simulink model "Model_plane2_Oldvers"  (R2023b)
settings: Solver=VariableStepAuto  StartTime=0.0  StopTime=5.0  RelTol=1e-3
values from neighbouring files (symbols this model uses):
  a_table = [340.3 339.5 338.8 338.0 337.2 336.4]    [Table1.m]
  Alfa = [-2 4 10 16]    [Table1.m]
  Alfa_table = [-4 0 5 10 20]    [Table1.m]
  Alfa_y = [-4 6 8 9 10 12 14]    [Table1.m]
  Cxa_table = [0.03434 0.0358 0.04274 ... (first row only)    [Table1.m]
  Cy_DB = [0.01242 0.01286 0.01457]    [Table1.m]
  Cy_fi = [0.00623 0.00643 0.00626]    [Table1.m]
  Cya = [-0.276 -0.330 -0.390 ... (first row only)    [Table1.m]
  H = [339 3256 4060 8000 12000]    [Table1.m]
  H_table = 0:2000:10000    [Table1.m]
  M_C = [0.4 0.6 0.82]    [Table1.m]
  M_mz = [0.2 0.4 0.6 0.8]    [Table1.m]
  M_mz2 = [0.4 0.7 0.85]    [Table1.m]
  M_table = [0.4 0.7 0.82]    [Table1.m]
  M_y = [0.4 0.7 0.82]    [Table1.m]
  mz_alfa = [-0.0282 -0.0282 -0.0289 -0.0404]    [Table1.m]
  mz_alfa2 = [-8.163 -8.762 -9.714 ... (first row only)    [Table1.m]
  mz_DB = [-0.0350 -0.0358 -0.0370 -0.0377]    [Table1.m]
  mz_fi = [-0.0695 -0.0714 -0.0739 -0.0832]    [Table1.m]
  mz_omz = [-23.768 -25.300 -28.284 ... (first row only)    [Table1.m]
  P = [9088 7396 6783 5000 4000]    [Table1.m]
  q_table = [1.225 1.2017 1.1786 1.1560 1.1337 1.1117]    [Table1.m]
libraries: simulink x2
settings Model: Creator=Анастасия  LastModifiedBy=Анастасия
settings RTWCC: GPUComputeCapability=5.0

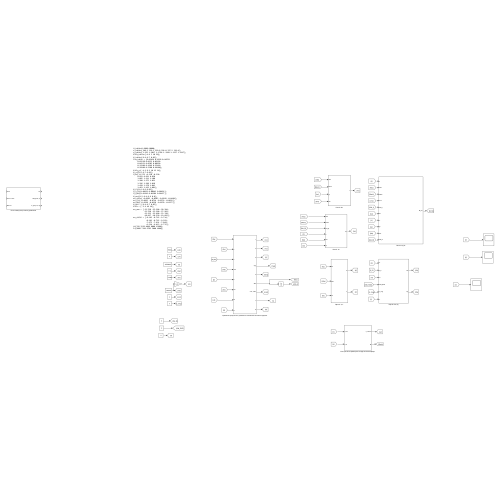
[thumbnail: Simulink's stored preview of the top-level diagram]
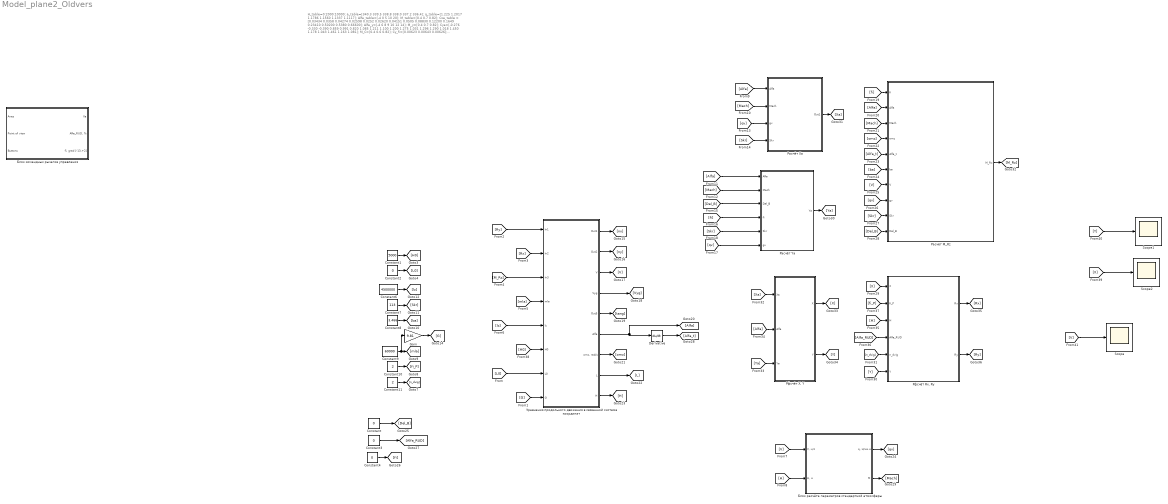
== system Model_plane2_Oldvers ==
  note: H_table=0:2000:10000;
      | a_table=[340.3 339.5 338.8 338.0 337.2 336.4];
      | q_table=[1.225 1.2017 1.1786 1.1560 1.1337 1.1117];
      | Alfa_table=[-4 0 5 10 20];
      | M_table=[0.4 0.7 0.82];
      | Cxa_table = [0.03434 0.0358 0.04274
      | 0.02598 0.0252 0.02620
      | 0.04151 0.0505 0.08830
      | 0.12200 0.1649 0.23410
      | 0.50200 0.5380 0.66600];
      | Alfa_y=[-4 6 8 9 10 12 14];
      | M_y=[0.4 0.7 0.82];
      | Cya=[-0.276 -0.330 -0.390
      | 0.859 0.991 0.820
      | 1.085 1.211 1.100
      | 1.200 1.275 1.031
      | 1.296 1.290 1.018
      | 1.450 1.178 1.043
      | 1.461 1.163 1.081];
      | M_C=[0.4 0.6 0.82];
      | Cy_fi=[0.00623 0.00643 0.00626];
      | Cy_DB=[0.01242 0.01286 0.01457];
      | M_mz=[0.2 0.4 0.6 0.8];
      | mz_alfa=[-0.0282 -0.0282 -0.0289 -0.0404];
      | mz_fi=[-0.0695 -0.0714 -0.0739 -0.0832];
      | mz_DB=[-0.0350 -0.0358 -0.0370 -0.0377];
      | M_mz2 = [0.4 0.7 0.85];
      | Alfa = [-2 4 10 16];
      | mz_omz = [-23.768 -25.300 -28.284;
      | -23.768 -25.300 -27.903;
      | -23.222 -22.600 -23.320;
      | -18.967 -18.520 -19.601];
      | mz_alfa2 = [-8.163 -8.762 -9.714;
      | -8.163 -8.762 -9.583;
      | -7.975 -7.991 -7.868;
      | -6.514 -6.413 -6.732];
      | H=[339 3256 4060 8000 12000];
      | P=[9088 7396 6783 5000 4000];
  Constant{,2..4} (4 alike) : Constant  Value=0
  Constant1 : Constant  Value=5000
  Constant10 : Constant  Value=2
  Constant11 : Constant  Value=2
  Constant6 : Constant  Value=4500000
  Constant7 : Constant  Value=113
  Constant8 : Constant  Value=3.466
  Constant9 : Constant  Value=60000
  Derivative : Derivative
  Gain : Gain  Gain=9.81
  Scope : Scope
  Scope1 : Scope
  Scope2 : Scope
  Блок командных рычагов управления : Subsystem
  Блок расчёта параметров стандартной атмосферы : Subsystem
  Расчёт M_Rz : Subsystem
  Расчёт Xa : Subsystem
  Расчёт Ya : Subsystem
  "Рфсчёт Rx, Ry" : Subsystem
  "Рфсчёт X, Y" : Subsystem
  Уравнения продольного движения в связанной системе координат : Subsystem
  wires:
  Constant1/1 -> [H0]
  Constant2/1 -> [L0]
  Constant6/1 -> [lz]
  Constant7/1 -> [Skr]
  Constant8/1 -> [ba]
  Constant9/1 -> Gain/1, [mla]
  Constant10/1 -> [fi_P]
  Constant11/1 -> [n_dvig]
  Gain/1 -> [G]
  [Ry] -> Уравнения продольного движения в связанной системе координат/1(In1)
  [Rx] -> Уравнения продольного движения в связанной системе координат/2(In2)
  [M_Rz] -> Уравнения продольного движения в связанной системе координат/3(In3)
  [mla] -> Уравнения продольного движения в связанной системе координат/4(mla)
  [lz] -> Уравнения продольного движения в связанной системе координат/5(lz)
  Уравнения продольного движения в связанной системе координат/1(Out1) -> [nx]
  Уравнения продольного движения в связанной системе координат/2(Out2) -> [ny]
  Уравнения продольного движения в связанной системе координат/3(V) -> [V]
  Уравнения продольного движения в связанной системе координат/4(Vyg) -> [Vyg]
  Уравнения продольного движения в связанной системе координат/5(Out5) -> [tang]
  Уравнения продольного движения в связанной системе координат/6(Alfa) -> Derivative/1, [Alfa]
  Уравнения продольного движения в связанной системе координат/7("omz, rad/s") -> [omz]
  Уравнения продольного движения в связанной системе координат/8(L) -> [L]
  Уравнения продольного движения в связанной системе координат/9(H) -> [H]
  Derivative/1 -> [Alfa_t]
  [V] -> Блок расчёта параметров стандартной атмосферы/1("V, м/с")
  [H] -> Блок расчёта параметров стандартной атмосферы/2("H, м")
  Блок расчёта параметров стандартной атмосферы/1("q, Н/кв.м") -> [qv]
  Блок расчёта параметров стандартной атмосферы/2(М) -> [Mach]
  [Alfa] -> Расчёт Xa/1(Alfa)
  [Mach] -> Расчёт Xa/2(Mach)
  [Mach] -> Расчёт Ya/2(Mach)
  [Alfa] -> Расчёт Ya/1(Alfa)
  Расчёт Xa/1(Out1) -> [Xa]
  Расчёт Ya/1(Ya) -> [Ya]
  [Skr] -> Расчёт Xa/4(Skr)
  [qv] -> Расчёт Xa/3(gv)
  [Del_B] -> Расчёт Ya/3(Del_B)
  [fi] -> Расчёт Ya/4(fi)
  [qv] -> Расчёт Ya/6(gv)
  [Skr] -> Расчёт Ya/5(Skr)
  Расчёт M_Rz/1(M_Rz) -> [M_Rz]
  [fi] -> Расчёт M_Rz/1(fi)
  [Alfa] -> Расчёт M_Rz/2(Alfa)
  [omz] -> Расчёт M_Rz/4(omz)
  [Mach] -> Расчёт M_Rz/3(Mach)
  [Alfa_t] -> Расчёт M_Rz/5(Alfa_t)
  [ba] -> Расчёт M_Rz/6(ba)
  [qv] -> Расчёт M_Rz/8(gv)
  [Del_B] -> Расчёт M_Rz/10(Del_B)
  [Skr] -> Расчёт M_Rz/9(Skr)
  [V] -> Расчёт M_Rz/7(V)
  "Рфсчёт X, Y"/1(X) -> [X]
  "Рфсчёт X, Y"/2(Y) -> [Y]
  [X] -> "Рфсчёт Rx, Ry"/1(X)
  [Y] -> "Рфсчёт Rx, Ry"/6(Y)
  "Рфсчёт Rx, Ry"/1(Rx) -> [Rx]
  "Рфсчёт Rx, Ry"/2(Ry) -> [Ry]
  [Xa] -> "Рфсчёт X, Y"/1(Xa)
  [Ya] -> "Рфсчёт X, Y"/3(Ya)
  [Alfa] -> "Рфсчёт X, Y"/2(Alfa)
  [Alfa_RUD] -> "Рфсчёт Rx, Ry"/4(Alfa_RUD)
  [n_dvig] -> "Рфсчёт Rx, Ry"/5(n_dvig)
  [H] -> "Рфсчёт Rx, Ry"/3(H)
  [fi_P] -> "Рфсчёт Rx, Ry"/2(fi_P)
  [H0] -> Уравнения продольного движения в связанной системе координат/6(H0)
  [L0] -> Уравнения продольного движения в связанной системе координат/7(L0)
  [G] -> Уравнения продольного движения в связанной системе координат/8(G)
  [V] -> Scope/1
  Constant4/1 -> [fi]
  Constant3/1 -> [Alfa_RUD]
  Constant/1 -> [Del_B]
  [Y] -> Scope1/1
  [X] -> Scope2/1

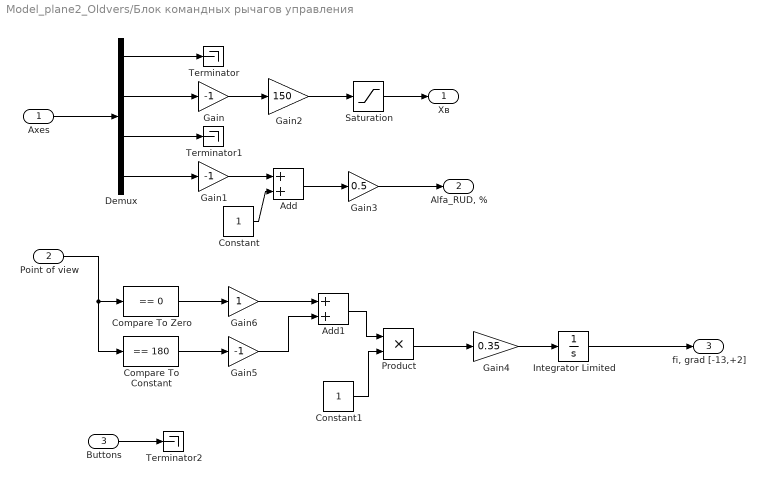
== system Model_plane2_Oldvers/Блок командных рычагов управления ==
  Axes : Inport
  Point of view : Inport  Port=2
  Buttons : Inport  Port=3
  Add : Sum
  Add1 : Sum
  Compare To Constant : simulink/Logic and Bit Operations/Compare To Constant  relop===  const=180  OutDataTypeStr=boolean
  Compare To Zero : simulink/Logic and Bit Operations/Compare To Zero  relop===  OutDataTypeStr=boolean
  Constant : Constant
  Constant1 : Constant
  Demux : Demux
  Gain : Gain  Gain=-1
  Gain1 : Gain  Gain=-1
  Gain2 : Gain  Gain=150
  Gain3 : Gain  Gain=0.5
  Gain4 : Gain  Gain=0.35
  Gain5 : Gain  Gain=-1
  Gain6 : Gain
  Integrator Limited : Integrator  LimitOutput=on  UpperSaturationLimit=1  LowerSaturationLimit=0
  Product : Product
  Saturation : Saturate
  Terminator : Terminator
  Terminator1 : Terminator
  Terminator2 : Terminator
  Xв : Outport
  "Alfa_RUD, %" : Outport  Port=2
  "fi, grad [-13,+2]" : Outport  Port=3
  wires:
  Axes/1 -> Demux/1
  Demux/1 -> Terminator/1
  Demux/3 -> Terminator1/1
  Demux/2 -> Gain/1
  Gain/1 -> Gain2/1
  Gain2/1 -> Saturation/1
  Saturation/1 -> Xв/1
  Demux/4 -> Gain1/1
  Gain1/1 -> Add/1
  Constant/1 -> Add/2
  Add/1 -> Gain3/1
  Gain3/1 -> "Alfa_RUD, %"/1
  Integrator Limited/1 -> "fi, grad [-13,+2]"/1
  Gain4/1 -> Integrator Limited/1
  Product/1 -> Gain4/1
  Constant1/1 -> Product/2
  Add1/1 -> Product/1
  Gain5/1 -> Add1/2
  Gain6/1 -> Add1/1
  Compare To Zero/1 -> Gain6/1
  Compare To Constant/1 -> Gain5/1
  Point of view/1 -> Compare To Constant/1, Compare To Zero/1
  Buttons/1 -> Terminator2/1

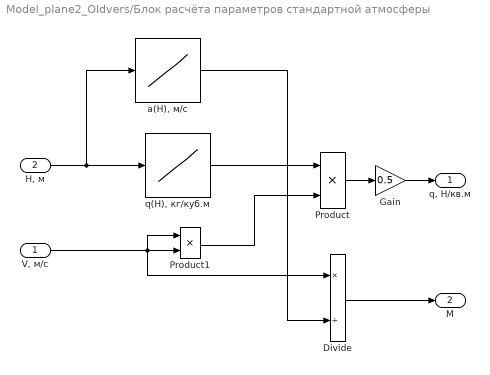
== system Model_plane2_Oldvers/Блок расчёта параметров стандартной атмосферы ==
  "V, м/с" : Inport
  "H, м" : Inport  Port=2
  Divide : Product  Inputs=*/
  Gain : Gain  Gain=0.5
  Product : Product
  Product1 : Product
  "a(H), м/с" : Lookup_n-D  NumberOfTableDimensions=1  BreakpointsForDimension1=H_table  Table=a_table  InternalRulePriority=Speed  RndMeth=Simplest
  "q(H), кг/куб.м" : Lookup_n-D  NumberOfTableDimensions=1  BreakpointsForDimension1=H_table  Table=q_table  InternalRulePriority=Speed  RndMeth=Simplest
  "q, Н/кв.м" : Outport
  М : Outport  Port=2
  wires:
  Gain/1 -> "q, Н/кв.м"/1
  "H, м"/1 -> "a(H), м/с"/1, "q(H), кг/куб.м"/1
  Product1/1 -> Product/2
  "V, м/с"/1 -> Divide/1, Product1/1, Product1/2
  "q(H), кг/куб.м"/1 -> Product/1
  "a(H), м/с"/1 -> Divide/2
  Product/1 -> Gain/1
  Divide/1 -> М/1

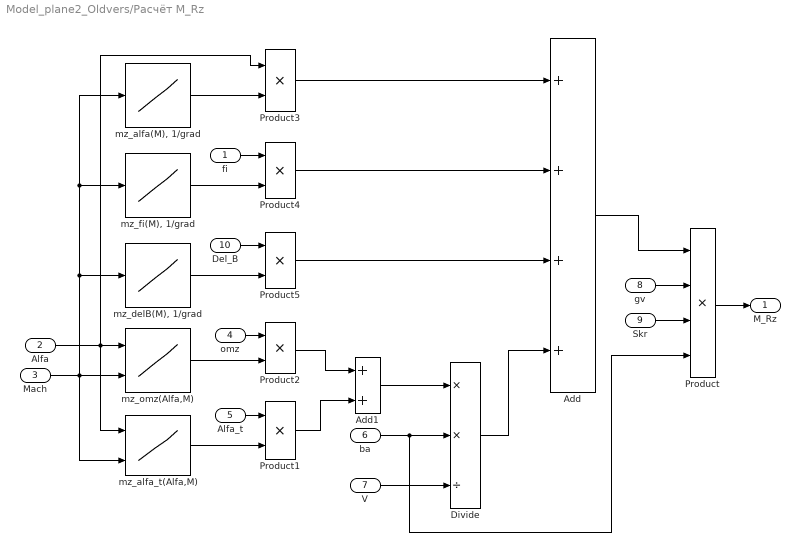
== system Model_plane2_Oldvers/Расчёт M_Rz ==
  fi : Inport
  Alfa : Inport  Port=2
  Mach : Inport  Port=3
  omz : Inport  Port=4
  Alfa_t : Inport  Port=5
  ba : Inport  Port=6
  V : Inport  Port=7
  gv : Inport  Port=8
  Skr : Inport  Port=9
  Del_B : Inport  Port=10
  Add : Sum  Inputs=++++
  Add1 : Sum
  Divide : Product  Inputs=**/
  Product : Product  Inputs=4
  Product{1..5} (5 alike) : Product
  "mz_alfa(M), 1/grad" : Lookup_n-D  NumberOfTableDimensions=1  BreakpointsForDimension1=M_mz  Table=mz_alfa  InternalRulePriority=Speed  RndMeth=Simplest
  mz_alfa_t(Alfa,M) : Lookup_n-D  BreakpointsForDimension1=Alfa  BreakpointsForDimension2=M_mz2  Table=mz_alfa2  InternalRulePriority=Speed  RndMeth=Simplest
      settings: InputPortMap=u0,u1
  "mz_delB(M), 1/grad" : Lookup_n-D  NumberOfTableDimensions=1  BreakpointsForDimension1=M_mz  Table=mz_DB  InternalRulePriority=Speed  RndMeth=Simplest
  "mz_fi(M), 1/grad" : Lookup_n-D  NumberOfTableDimensions=1  BreakpointsForDimension1=M_mz  Table=mz_fi  InternalRulePriority=Speed  RndMeth=Simplest
  mz_omz(Alfa,M) : Lookup_n-D  BreakpointsForDimension1=Alfa  BreakpointsForDimension2=M_mz2  Table=mz_omz  InternalRulePriority=Speed  RndMeth=Simplest
      settings: InputPortMap=u0,u1
  M_Rz : Outport
  wires:
  fi/1 -> Product4/1
  Product/1 -> M_Rz/1
  ba/1 -> Product/4, Divide/2
  Skr/1 -> Product/3
  gv/1 -> Product/2
  Add/1 -> Product/1
  V/1 -> Divide/3
  Divide/1 -> Add/4
  Add1/1 -> Divide/1
  Product2/1 -> Add1/1
  Product1/1 -> Add1/2
  Alfa_t/1 -> Product1/1
  omz/1 -> Product2/1
  mz_omz(Alfa,M)/1 -> Product2/2
  mz_alfa_t(Alfa,M)/1 -> Product1/2
  Alfa/1 -> mz_omz(Alfa,M)/1, mz_alfa_t(Alfa,M)/1, Product3/1
  Mach/1 -> mz_omz(Alfa,M)/2, "mz_alfa(M), 1/grad"/1, "mz_fi(M), 1/grad"/1, "mz_delB(M), 1/grad"/1, mz_alfa_t(Alfa,M)/2
  "mz_alfa(M), 1/grad"/1 -> Product3/2
  "mz_fi(M), 1/grad"/1 -> Product4/2
  "mz_delB(M), 1/grad"/1 -> Product5/2
  Del_B/1 -> Product5/1
  Product3/1 -> Add/1
  Product4/1 -> Add/2
  Product5/1 -> Add/3

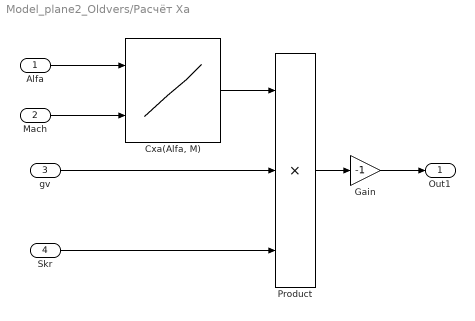
== system Model_plane2_Oldvers/Расчёт Xa ==
  Alfa : Inport
  Mach : Inport  Port=2
  gv : Inport  Port=3
  Skr : Inport  Port=4
  "Cxa(Alfa, M)" : Lookup_n-D  BreakpointsForDimension1=Alfa_table  BreakpointsForDimension2=M_table  Table=Cxa_table  InternalRulePriority=Speed  RndMeth=Simplest
      settings: InputPortMap=u0,u1
  Gain : Gain  Gain=-1
  Product : Product  Inputs=3
  Out1 : Outport
  wires:
  Alfa/1 -> "Cxa(Alfa, M)"/1
  Product/1 -> Gain/1
  Gain/1 -> Out1/1
  Skr/1 -> Product/3
  gv/1 -> Product/2
  Mach/1 -> "Cxa(Alfa, M)"/2
  "Cxa(Alfa, M)"/1 -> Product/1

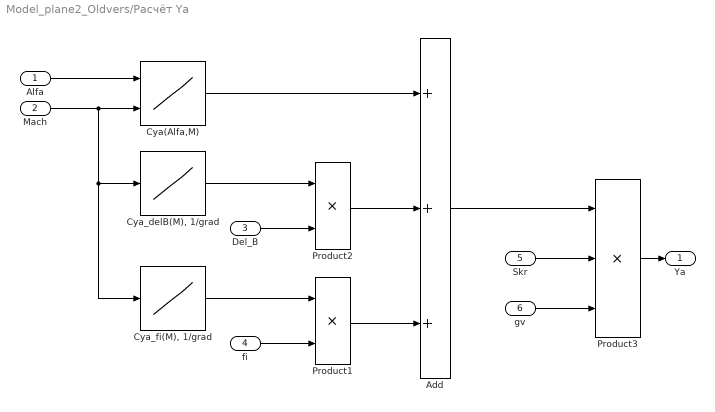
== system Model_plane2_Oldvers/Расчёт Ya ==
  Alfa : Inport
  Mach : Inport  Port=2
  Del_B : Inport  Port=3
  fi : Inport  Port=4
  Skr : Inport  Port=5
  gv : Inport  Port=6
  Add : Sum  Inputs=+++
  Cya(Alfa,M) : Lookup_n-D  BreakpointsForDimension1=Alfa_y  BreakpointsForDimension2=M_y  Table=Cya  InternalRulePriority=Speed  RndMeth=Simplest
      settings: InputPortMap=u0,u1
  "Cya_delB(M), 1/grad" : Lookup_n-D  NumberOfTableDimensions=1  BreakpointsForDimension1=M_C  Table=Cy_DB  InternalRulePriority=Speed  RndMeth=Simplest
  "Cya_fi(M), 1/grad" : Lookup_n-D  NumberOfTableDimensions=1  BreakpointsForDimension1=M_C  Table=Cy_fi  InternalRulePriority=Speed  RndMeth=Simplest
  Product1 : Product
  Product2 : Product
  Product3 : Product  Inputs=3
  Ya : Outport
  wires:
  Alfa/1 -> Cya(Alfa,M)/1
  fi/1 -> Product1/2
  Del_B/1 -> Product2/2
  gv/1 -> Product3/3
  Skr/1 -> Product3/2
  Product3/1 -> Ya/1
  "Cya_fi(M), 1/grad"/1 -> Product1/1
  "Cya_delB(M), 1/grad"/1 -> Product2/1
  Mach/1 -> "Cya_delB(M), 1/grad"/1, "Cya_fi(M), 1/grad"/1, Cya(Alfa,M)/2
  Cya(Alfa,M)/1 -> Add/1
  Product2/1 -> Add/2
  Product1/1 -> Add/3
  Add/1 -> Product3/1

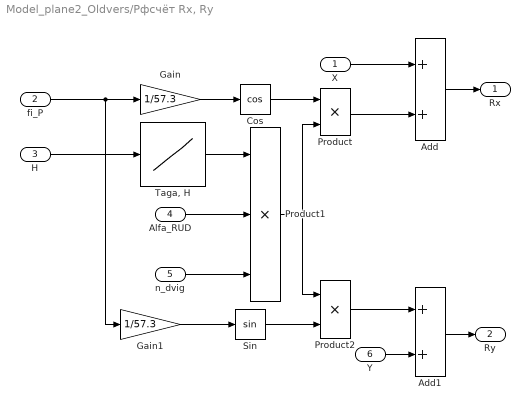
== system Model_plane2_Oldvers/Рфсчёт Rx, Ry ==
  X : Inport
  fi_P : Inport  Port=2
  H : Inport  Port=3
  Alfa_RUD : Inport  Port=4
  n_dvig : Inport  Port=5
  Y : Inport  Port=6
  Add : Sum
  Add1 : Sum
  Cos : Trigonometry  Operator=cos
  Gain : Gain  Gain=1/57.3
  Gain1 : Gain  Gain=1/57.3
  Product : Product
  Product1 : Product  Inputs=3
  Product2 : Product
  Sin : Trigonometry
  "Taga, H" : Lookup_n-D  NumberOfTableDimensions=1  BreakpointsForDimension1=H  Table=P  InternalRulePriority=Speed  RndMeth=Simplest
  Rx : Outport
  Ry : Outport  Port=2
  wires:
  X/1 -> Add/1
  Product/1 -> Add/2
  Cos/1 -> Product/1
  Gain/1 -> Cos/1
  fi_P/1 -> Gain/1, Gain1/1
  "Taga, H"/1 -> Product1/1
  Alfa_RUD/1 -> Product1/2
  n_dvig/1 -> Product1/3
  H/1 -> "Taga, H"/1
  Product1/1 -> Product/2, Product2/1
  Sin/1 -> Product2/2
  Gain1/1 -> Sin/1
  Add/1 -> Rx/1
  Product2/1 -> Add1/1
  Y/1 -> Add1/2
  Add1/1 -> Ry/1

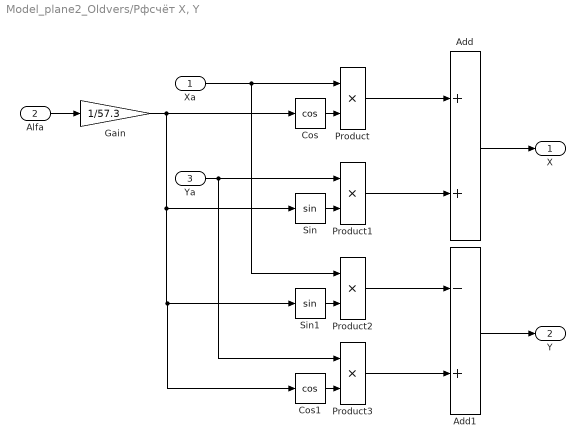
== system Model_plane2_Oldvers/Рфсчёт X, Y ==
  Xa : Inport
  Alfa : Inport  Port=2
  Ya : Inport  Port=3
  Add : Sum
  Add1 : Sum  Inputs=-+
  Cos : Trigonometry  Operator=cos
  Cos1 : Trigonometry  Operator=cos
  Gain : Gain  Gain=1/57.3
  Product{,1..3} (4 alike) : Product
  Sin : Trigonometry
  Sin1 : Trigonometry
  X : Outport
  Y : Outport  Port=2
  wires:
  Xa/1 -> Product2/1, Product/1
  Cos/1 -> Product/2
  Gain/1 -> Cos1/1, Sin1/1, Sin/1, Cos/1
  Alfa/1 -> Gain/1
  Ya/1 -> Product3/1, Product1/1
  Sin/1 -> Product1/2
  Sin1/1 -> Product2/2
  Cos1/1 -> Product3/2
  Product/1 -> Add/1
  Product1/1 -> Add/2
  Product2/1 -> Add1/1
  Product3/1 -> Add1/2
  Add/1 -> X/1
  Add1/1 -> Y/1

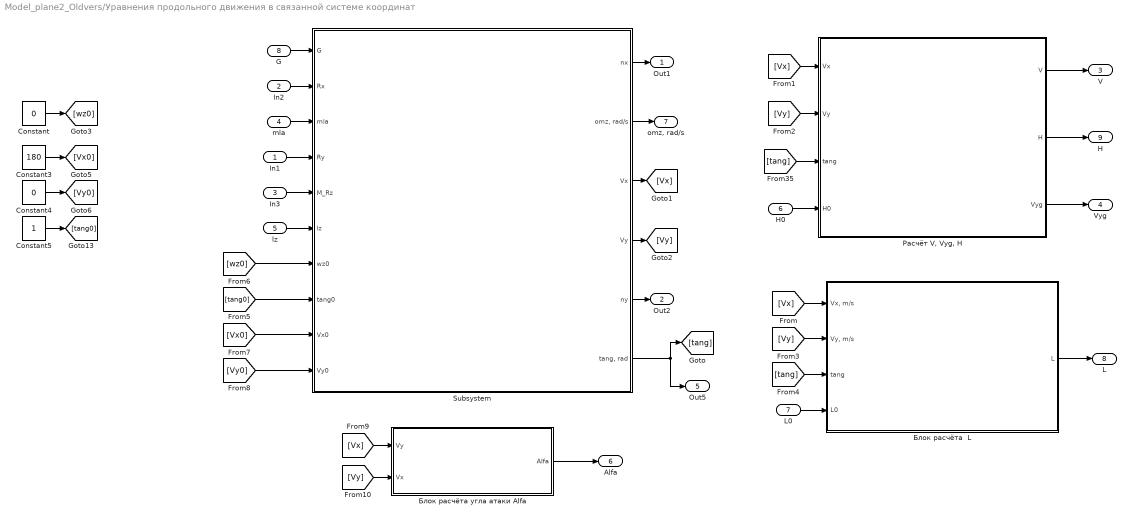
== system Model_plane2_Oldvers/Уравнения продольного движения в связанной системе координат ==
  In1 : Inport
  In2 : Inport  Port=2
  In3 : Inport  Port=3
  mla : Inport  Port=4
  lz : Inport  Port=5
  H0 : Inport  Port=6
  L0 : Inport  Port=7
  G : Inport  Port=8
  Constant : Constant  Value=0
  Constant3 : Constant  Value=180
  Constant4 : Constant  Value=0
  Constant5 : Constant
  Subsystem : Subsystem
  Блок расчёта  L : Subsystem
  Блок расчёта угла атаки Alfa : Subsystem
  "Расчёт V, Vyg, H" : Subsystem
  Out1 : Outport
  Out2 : Outport  Port=2
  V : Outport  Port=3
  Vyg : Outport  Port=4
  Out5 : Outport  Port=5
  Alfa : Outport  Port=6
  "omz, rad/s" : Outport  Port=7
  L : Outport  Port=8
  H : Outport  Port=9
  wires:
  [tang] -> "Расчёт V, Vyg, H"/3(tang)
  "Расчёт V, Vyg, H"/2(H) -> H/1
  "Расчёт V, Vyg, H"/3(Vyg) -> Vyg/1
  "Расчёт V, Vyg, H"/1(V) -> V/1
  H0/1 -> "Расчёт V, Vyg, H"/4(H0)
  Блок расчёта  L/1(L) -> L/1
  Subsystem/1(nx) -> Out1/1
  Subsystem/5(ny) -> Out2/1
  Subsystem/6("tang, rad") -> Out5/1, [tang]
  [Vx] -> "Расчёт V, Vyg, H"/1(Vx)
  [Vy] -> "Расчёт V, Vyg, H"/2(Vy)
  Subsystem/3(Vx) -> [Vx]
  Subsystem/4(Vy) -> [Vy]
  Subsystem/2("omz, rad/s") -> "omz, rad/s"/1
  [Vx] -> Блок расчёта  L/1("Vx, m/s")
  [Vy] -> Блок расчёта  L/2("Vy, m/s")
  [tang] -> Блок расчёта  L/3(tang)
  L0/1 -> Блок расчёта  L/4(L0)
  G/1 -> Subsystem/1(G)
  In2/1 -> Subsystem/2(Rx)
  In1/1 -> Subsystem/4(Ry)
  In3/1 -> Subsystem/5(M_Rz)
  lz/1 -> Subsystem/6(lz)
  Constant5/1 -> [tang0]
  Constant4/1 -> [Vy0]
  Constant3/1 -> [Vx0]
  Constant/1 -> [wz0]
  [tang0] -> Subsystem/8(tang0)
  [wz0] -> Subsystem/7(wz0)
  [Vx0] -> Subsystem/9(Vx0)
  [Vy0] -> Subsystem/10(Vy0)
  mla/1 -> Subsystem/3(mla)
  Блок расчёта угла атаки Alfa/1(Alfa) -> Alfa/1
  [Vx] -> Блок расчёта угла атаки Alfa/1(Vy)
  [Vy] -> Блок расчёта угла атаки Alfa/2(Vx)

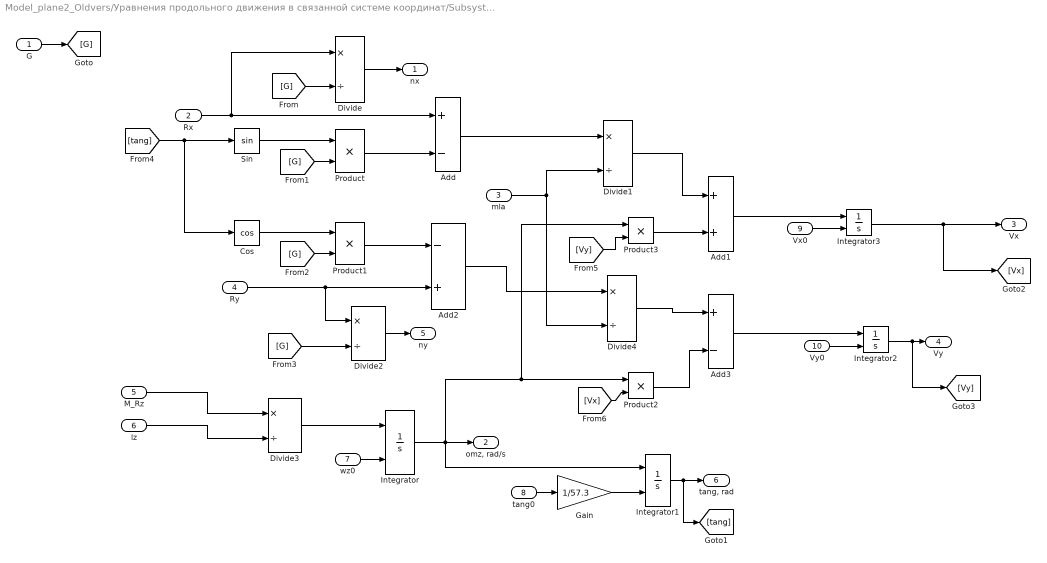
== system Model_plane2_Oldvers/Уравнения продольного движения в связанной системе координат/Subsystem ==
  G : Inport
  Rx : Inport  Port=2
  mla : Inport  Port=3
  Ry : Inport  Port=4
  M_Rz : Inport  Port=5
  lz : Inport  Port=6
  wz0 : Inport  Port=7
  tang0 : Inport  Port=8
  Vx0 : Inport  Port=9
  Vy0 : Inport  Port=10
  Add : Sum  Inputs=+-
  Add1 : Sum
  Add2 : Sum  Inputs=-+
  Add3 : Sum  Inputs=+-
  Cos : Trigonometry  Operator=cos
  Divide{,1..4} (5 alike) : Product  Inputs=*/
  Gain : Gain  Gain=1/57.3
  Integrator{,1..3} (4 alike) : Integrator  InitialConditionSource=external
  Product{,1..3} (4 alike) : Product
  Sin : Trigonometry
  nx : Outport
  "omz, rad/s" : Outport  Port=2
  Vx : Outport  Port=3
  Vy : Outport  Port=4
  ny : Outport  Port=5
  "tang, rad" : Outport  Port=6
  wires:
  G/1 -> [G]
  Rx/1 -> Divide/1, Add/1
  Product/1 -> Add/2
  [G] -> Divide/2
  [G] -> Product/2
  Sin/1 -> Product/1
  [tang] -> Cos/1, Sin/1
  Divide/1 -> nx/1
  Add/1 -> Divide1/1
  mla/1 -> Divide4/2, Divide1/2
  Cos/1 -> Product1/1
  [G] -> Product1/2
  Product1/1 -> Add2/1
  Ry/1 -> Divide2/1, Add2/2
  [G] -> Divide2/2
  Divide2/1 -> ny/1
  M_Rz/1 -> Divide3/1
  lz/1 -> Divide3/2
  wz0/1 -> Integrator/2
  Divide3/1 -> Integrator/1
  Integrator/1 -> Integrator1/1, Product3/1, Product2/1, "omz, rad/s"/1
  Add2/1 -> Divide4/1
  Divide4/1 -> Add3/1
  Product2/1 -> Add3/2
  tang0/1 -> Gain/1
  Gain/1 -> Integrator1/2
  Add3/1 -> Integrator2/1
  Vx0/1 -> Integrator3/2
  Add1/1 -> Integrator3/1
  Divide1/1 -> Add1/1
  Product3/1 -> Add1/2
  Vy0/1 -> Integrator2/2
  Integrator3/1 -> [Vx], Vx/1
  Integrator2/1 -> [Vy], Vy/1
  Integrator1/1 -> [tang], "tang, rad"/1
  [Vy] -> Product3/2
  [Vx] -> Product2/2

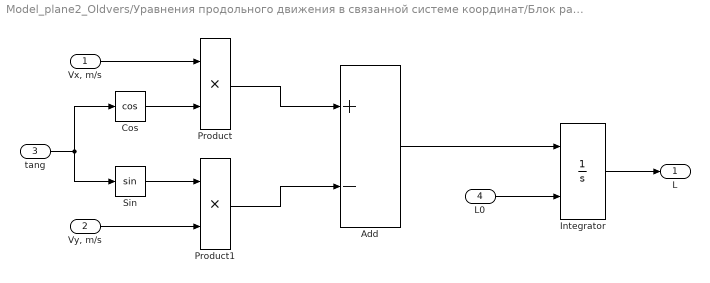
== system Model_plane2_Oldvers/Уравнения продольного движения в связанной системе координат/Блок расчёта  L ==
  "Vx, m/s" : Inport
  "Vy, m/s" : Inport  Port=2
  tang : Inport  Port=3
  L0 : Inport  Port=4
  Add : Sum  Inputs=+-
  Cos : Trigonometry  Operator=cos
  Integrator : Integrator  InitialConditionSource=external
  Product : Product
  Product1 : Product
  Sin : Trigonometry
  L : Outport
  wires:
  "Vx, m/s"/1 -> Product/1
  tang/1 -> Sin/1, Cos/1
  Cos/1 -> Product/2
  Sin/1 -> Product1/1
  "Vy, m/s"/1 -> Product1/2
  Product/1 -> Add/1
  Product1/1 -> Add/2
  L0/1 -> Integrator/2
  Add/1 -> Integrator/1
  Integrator/1 -> L/1

== system Model_plane2_Oldvers/Уравнения продольного движения в связанной системе координат/Блок расчёта угла атаки Alfa ==
  Vy : Inport
  Vx : Inport  Port=2
  Atan : Trigonometry  Operator=atan
  Divide : Product  Inputs=*/
  Gain : Gain  Gain=57.3
  Gain1 : Gain  Gain=57.3
  Alfa : Outport
  wires:
  Vy/1 -> Divide/1
  Vx/1 -> Divide/2
  Divide/1 -> Gain/1
  Gain/1 -> Atan/1
  Atan/1 -> Gain1/1
  Gain1/1 -> Alfa/1

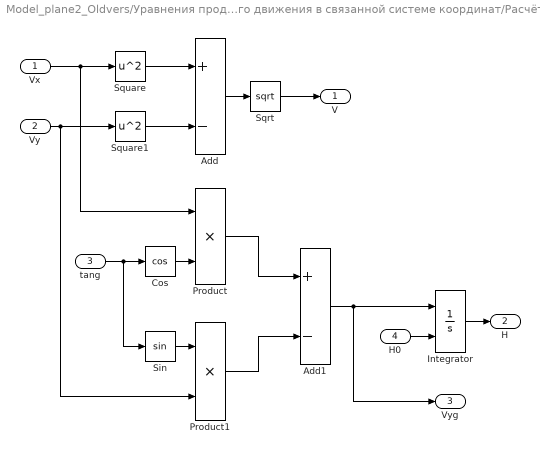
== system Model_plane2_Oldvers/Уравнения продольного движения в связанной системе координат/Расчёт V, Vyg, H ==
  Vx : Inport
  Vy : Inport  Port=2
  tang : Inport  Port=3
  H0 : Inport  Port=4
  Add : Sum  Inputs=+-
  Add1 : Sum  Inputs=+-
  Cos : Trigonometry  Operator=cos
  Integrator : Integrator  InitialConditionSource=external
  Product : Product
  Product1 : Product
  Sin : Trigonometry
  Sqrt : Sqrt  IntermediateResultsDataTypeStr=double
  Square : Math  Operator=square
  Square1 : Math  Operator=square
  V : Outport
  H : Outport  Port=2
  Vyg : Outport  Port=3
  wires:
  Vx/1 -> Square/1, Product/1
  Vy/1 -> Square1/1, Product1/2
  Square/1 -> Add/1
  Square1/1 -> Add/2
  Add/1 -> Sqrt/1
  Sqrt/1 -> V/1
  Cos/1 -> Product/2
  Sin/1 -> Product1/1
  tang/1 -> Cos/1, Sin/1
  Product/1 -> Add1/1
  Product1/1 -> Add1/2
  H0/1 -> Integrator/2
  Add1/1 -> Vyg/1, Integrator/1
  Integrator/1 -> H/1
